simulink model "ACC_sl"  (R2020b)
settings: Solver=ode4  StartTime=0.0  StopTime=500  FixedStep=0.01  RelTol=1e-3
values from neighbouring files (symbols this model uses):
  d0 = 5    [ACC_m.m]
  K1 = K(1)    [ACC_m.m]
  K2 = K(2)    [ACC_m.m]
  K3 = K(3)    [ACC_m.m]
  K4 = K(4)    [ACC_m.m]
  v0 = 0.1933    [ACC_m.m]    (also in identificacion.m)
undefined symbols (not defined in the file or in its folder): DiscIntNeverNeededParam
libraries: simulink x1
settings Model: Creator=pcx  LastModifiedBy=pcx
settings DebuggingCC: SFMachineParentedDataDiag=error

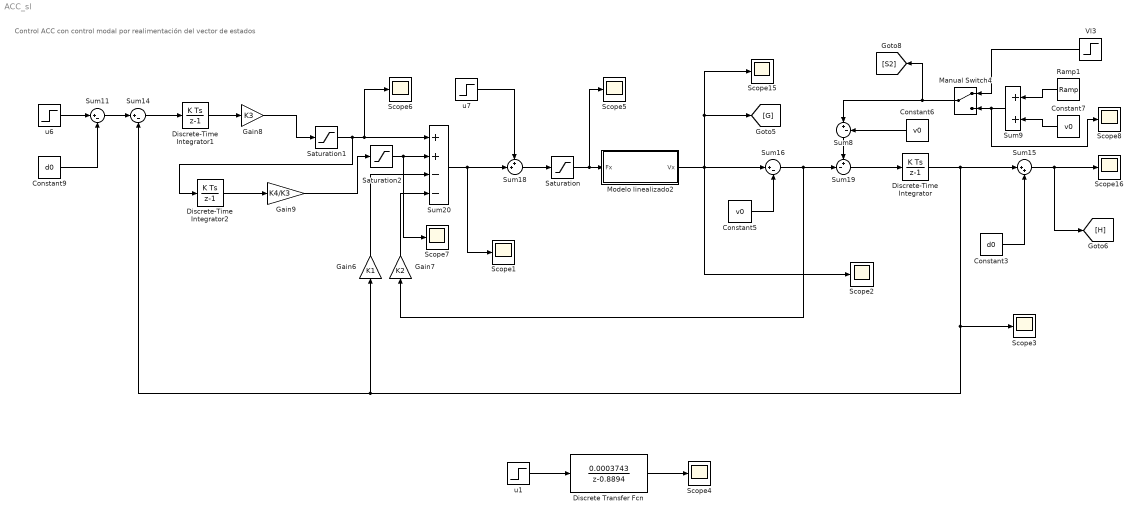
== system ACC_sl ==
  note: Control ACC con control modal por realimentación del vector de estados
  Constant3 : Constant  Value=d0
  Constant5 : Constant  Value=v0
  Constant6 : Constant  Value=v0
  Constant7 : Constant  Value=v0
  Constant9 : Constant  Value=d0
  Discrete Transfer Fcn : DiscreteTransferFcn  Numerator=[0.0003743]  Denominator=[1 -0.8894]  SampleTime=0.1
  Discrete-Time Integrator : DiscreteIntegrator  SampleTime=0.1  ICPrevOutput=DiscIntNeverNeededParam  ICPrevScaledInput=DiscIntNeverNeededParam
  Discrete-Time Integrator1 : DiscreteIntegrator  SampleTime=0.1  ICPrevOutput=DiscIntNeverNeededParam  ICPrevScaledInput=DiscIntNeverNeededParam
  Discrete-Time Integrator2 : DiscreteIntegrator  SampleTime=0.1  ICPrevOutput=DiscIntNeverNeededParam  ICPrevScaledInput=DiscIntNeverNeededParam
  Gain6 : Gain  Gain=K1
  Gain7 : Gain  Gain=K2
  Gain8 : Gain  Gain=K3
  Gain9 : Gain  Gain=K4/K3
  Manual Switch4 : ManualSwitch
  Modelo linealizado2 : Subsystem
      mask Display:
      | disp('Modelo \n linealizado')
      | port_label('input',1,'u')
      | port_label('output',1,'y')
  Ramp1 : simulink/Sources/Ramp  slope=0.01  start=10  InitialOutput=0
  Saturation : Saturate  UpperLimit=135  LowerLimit=0
  Saturation1 : Saturate  UpperLimit=250  LowerLimit=-inf
  Saturation2 : Saturate  UpperLimit=350  LowerLimit=-inf
  Scope{1..8,15..16} (10 alike) : Scope
  Sum{8,11,14,16} (4 alike) : Sum  Inputs=|+-
  Sum15 : Sum  Inputs=|++
  Sum18 : Sum  Inputs=++|
  Sum19 : Sum  Inputs=+-|
  Sum20 : Sum  Inputs=++--
  Sum9 : Sum
  Vl3 : Step  Time=20  Before=v0  After=v0+0.2  SampleTime=0.1
  u1 : Step  Time=0  SampleTime=0.01
  u6 : Step  Time=0  Before=5  After=5  SampleTime=0.1
  u7 : Step  Time=0  After=0  SampleTime=0
  wires:
  Constant6/1 -> Sum8/2
  Constant9/1 -> Sum11/2
  Sum11/1 -> Sum14/1
  Ramp1/1 -> Sum9/1
  Sum9/1 -> Scope8/1, Manual Switch4/2
  u6/1 -> Sum11/1
  Sum8/1 -> Sum19/1
  Vl3/1 -> Manual Switch4/1
  Modelo linealizado2/1(Vx) -> Sum16/1, [G], Scope15/1, Scope2/1
  Manual Switch4/1 -> [S2], Sum8/1
  u7/1 -> Sum18/1
  Gain9/1 -> Saturation2/1
  Sum20/1 -> Sum18/2, Scope1/1
  Constant7/1 -> Sum9/2
  Discrete-Time Integrator1/1 -> Gain8/1
  Discrete-Time Integrator/1 -> Sum15/1, Scope3/1, Gain6/1, Sum14/2
  Gain8/1 -> Saturation1/1
  Sum15/1 -> [H], Scope16/1
  Constant5/1 -> Sum16/2
  Constant3/1 -> Sum15/2
  Sum14/1 -> Discrete-Time Integrator1/1
  Discrete-Time Integrator2/1 -> Gain9/1
  Sum18/1 -> Saturation/1
  Saturation/1 -> Scope5/1, Modelo linealizado2/1(Fx)
  u1/1 -> Discrete Transfer Fcn/1
  Discrete Transfer Fcn/1 -> Scope4/1
  Sum16/1 -> Sum19/2, Gain7/1
  Sum19/1 -> Discrete-Time Integrator/1
  Gain6/1 -> Sum20/3
  Gain7/1 -> Sum20/4
  Saturation1/1 -> Discrete-Time Integrator2/1, Scope6/1, Sum20/1
  Saturation2/1 -> Scope7/1, Sum20/2

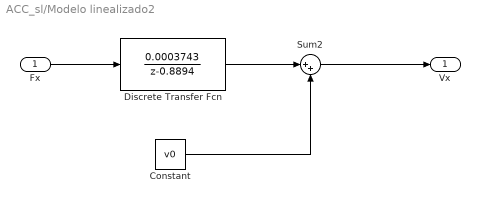
== system ACC_sl/Modelo linealizado2 ==
  Fx : Inport
  Constant : Constant  Value=v0
  Discrete Transfer Fcn : DiscreteTransferFcn  Numerator=[0.0003743]  Denominator=[1 -0.8894]  SampleTime=0.1
  Sum2 : Sum  Inputs=|++
  Vx : Outport
  wires:
  Fx/1 -> Discrete Transfer Fcn/1
  Sum2/1 -> Vx/1
  Discrete Transfer Fcn/1 -> Sum2/1
  Constant/1 -> Sum2/2
